simulink model "4pointDFT"  (R2021b)
settings: Solver=VariableStepAuto  StartTime=0.0  StopTime=10.0  RelTol=1e-3
undefined symbols (not defined in the file or in its folder): i
settings Model: Creator=Admin  LastModifiedBy=Admin

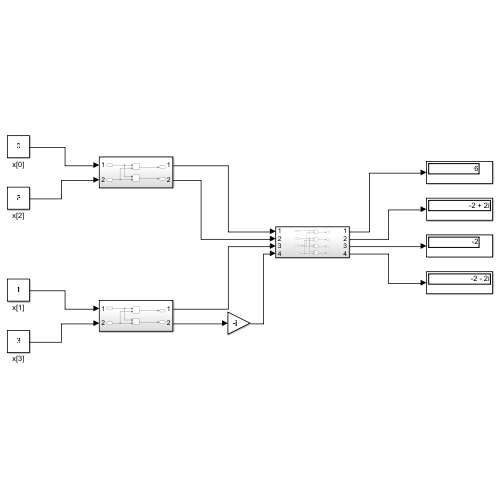
[thumbnail: Simulink's stored preview of the top-level diagram]
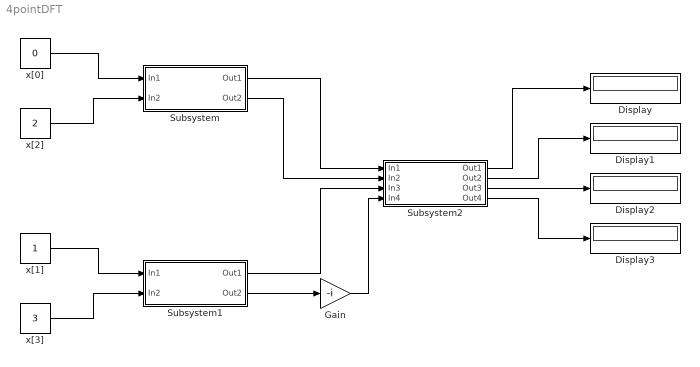
== system 4pointDFT ==
  Display{,1..3} (4 alike) : Display
  Gain : Gain  Gain=-i
  Subsystem : Subsystem
  Subsystem1 : Subsystem
  Subsystem2 : Subsystem
  x[0] : Constant  Value=0
  x[1] : Constant
  x[2] : Constant  Value=2
  x[3] : Constant  Value=3
  wires:
  Gain/1 -> Subsystem2/4(In4)
  Subsystem1/2(Out2) -> Gain/1
  x[3]/1 -> Subsystem1/2(In2)
  Subsystem1/1(Out1) -> Subsystem2/3(In3)
  x[1]/1 -> Subsystem1/1(In1)
  x[2]/1 -> Subsystem/2(In2)
  x[0]/1 -> Subsystem/1(In1)
  Subsystem/2(Out2) -> Subsystem2/2(In2)
  Subsystem/1(Out1) -> Subsystem2/1(In1)
  Subsystem2/4(Out4) -> Display3/1
  Subsystem2/3(Out3) -> Display2/1
  Subsystem2/2(Out2) -> Display1/1
  Subsystem2/1(Out1) -> Display/1

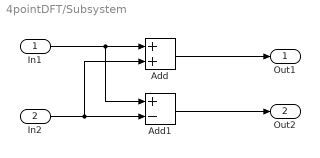
== system 4pointDFT/Subsystem ==
  In1 : Inport
  In2 : Inport  Port=2
  Add : Sum
  Add1 : Sum  Inputs=+-
  Out1 : Outport
  Out2 : Outport  Port=2
  wires:
  In1/1 -> Add1/1, Add/1
  In2/1 -> Add/2, Add1/2
  Add/1 -> Out1/1
  Add1/1 -> Out2/1

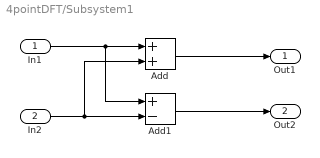
== system 4pointDFT/Subsystem1 ==
  In1 : Inport
  In2 : Inport  Port=2
  Add : Sum
  Add1 : Sum  Inputs=+-
  Out1 : Outport
  Out2 : Outport  Port=2
  wires:
  In1/1 -> Add1/1, Add/1
  In2/1 -> Add/2, Add1/2
  Add/1 -> Out1/1
  Add1/1 -> Out2/1

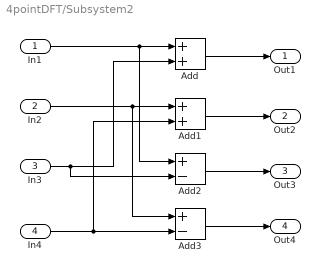
== system 4pointDFT/Subsystem2 ==
  In1 : Inport
  In2 : Inport  Port=2
  In3 : Inport  Port=3
  In4 : Inport  Port=4
  Add : Sum
  Add1 : Sum
  Add2 : Sum  Inputs=+-
  Add3 : Sum  Inputs=+-
  Out1 : Outport
  Out2 : Outport  Port=2
  Out3 : Outport  Port=3
  Out4 : Outport  Port=4
  wires:
  In1/1 -> Add2/1, Add/1
  Add/1 -> Out1/1
  In3/1 -> Add2/2, Add/2
  In2/1 -> Add3/1, Add1/1
  Add1/1 -> Out2/1
  Add3/1 -> Out4/1
  Add2/1 -> Out3/1
  In4/1 -> Add1/2, Add3/2
